simulink model "TesteDegrauMinQuadSimulinkX"  (R2015a)
settings: Solver=ode45  StartTime=0.0  StopTime=51  RelTol=1e-3
values from neighbouring files (symbols this model uses):
  T = 0.04    [Minimos_Quadrados.m]    (also in TesteDegrauMinQuad.m = 0.03)
  tf_digital_dnX = MinimosQuadrados(N, y, u, T, ordem)    [Minimos_Quadrados.m]
  tf_digital_dpX = MinimosQuadrados(N, y, u, T, ordem)    [Minimos_Quadrados.m]
  tf_digital_wnX = MinimosQuadrados(N, y, u, T, ordem)    [Minimos_Quadrados.m]
settings Model: Creator=Lucas  LastModifiedBy=Lucas

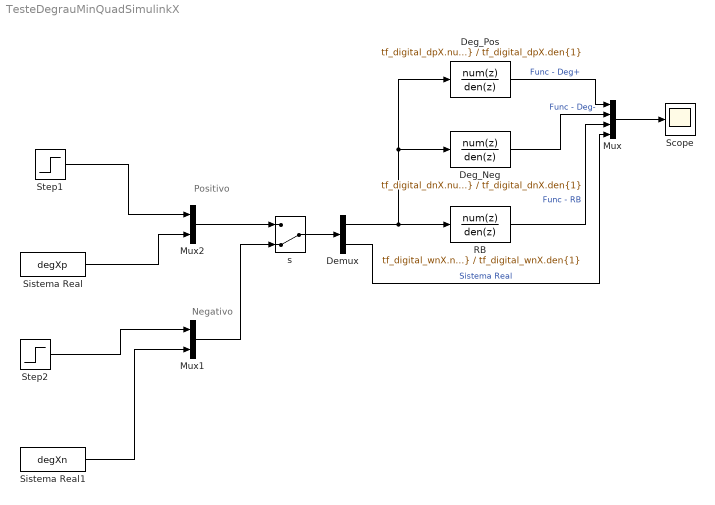
== system TesteDegrauMinQuadSimulinkX ==
  note: Positivo
  note: Negativo
  Deg_Neg : DiscreteTransferFcn  Numerator=tf_digital_dnX.num{1}  Denominator=tf_digital_dnX.den{1}  SampleTime=T
  Deg_Pos : DiscreteTransferFcn  Numerator=tf_digital_dpX.num{1}  Denominator=tf_digital_dpX.den{1}  SampleTime=T
  Demux : Demux  Outputs=2
  Mux : Mux
  Mux1 : Mux  Inputs=2
  Mux2 : Mux  Inputs=2
  RB : DiscreteTransferFcn  Numerator=tf_digital_wnX.num{1}  Denominator=tf_digital_wnX.den{1}  SampleTime=T
  Scope : Scope
      settings: ShowLegends=on
  Sistema Real : FromWorkspace  VariableName=degXp  SampleTime=0
  Sistema Real1 : FromWorkspace  VariableName=degXn  SampleTime=0
  Step1 : Step  Time=11  After=10  SampleTime=T
  Step2 : Step  Time=11  After=-10  SampleTime=T
  s : ManualSwitch  CurrentSetting=0
  wires:
  Deg_Pos/1 -> Mux/1  "Func - Deg+"
  Mux/1 -> Scope/1
  Deg_Neg/1 -> Mux/2  "Func - Deg-"
  RB/1 -> Mux/3  "Func - RB"
  s/1 -> Demux/1
  Sistema Real/1 -> Mux2/2
  Step1/1 -> Mux2/1
  Sistema Real1/1 -> Mux1/2
  Step2/1 -> Mux1/1
  Mux1/1 -> s/2
  Mux2/1 -> s/1
  Demux/1 -> Deg_Pos/1, Deg_Neg/1, RB/1
  Demux/2 -> Mux/4  "Sistema Real"
